simulink model "Project"  (R2019a)
settings: Solver=VariableStepAuto  StartTime=0.0  StopTime=9  RelTol=1e-3
model workspace (MAT data in the model file):
  tc = 0.05
libraries: Solver_SF x2, simulink x2
settings Model: Creator=admin  LastModifiedBy=Chuan
settings DataIOCC: ReturnWorkspaceOutputs=off

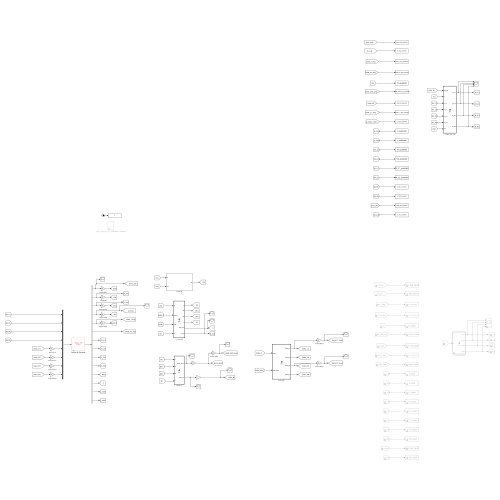
[thumbnail: Simulink's stored preview of the top-level diagram]
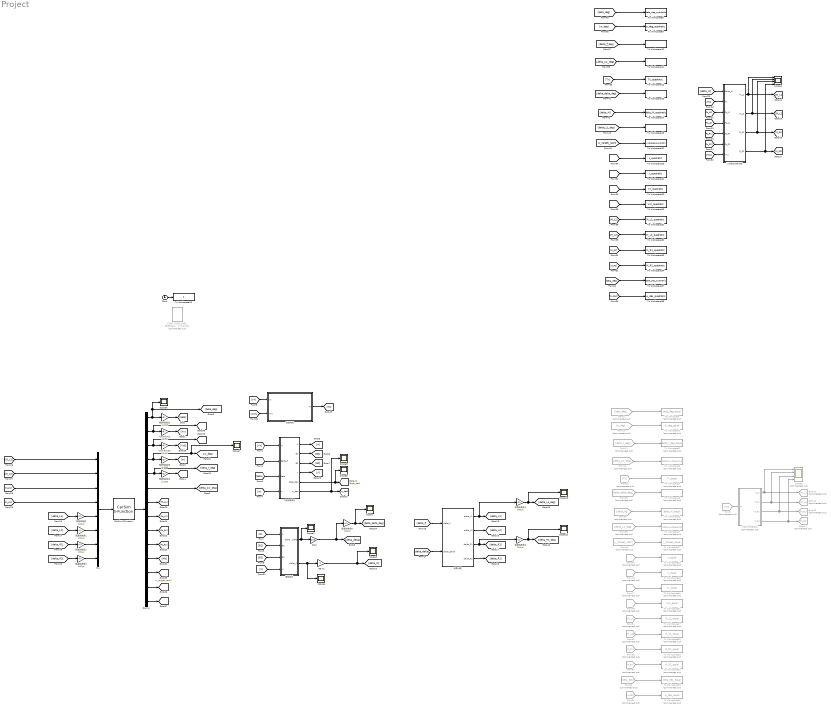
== system Project ==
  CarSim S-Function : Solver_SF/CarSim S-Function  Priority=1  SIMFILE=simfile.sim
  Clock : Clock
  Demux : Demux  Outputs=14
  From10 : From  Commented=on  GotoTag=w_deg
  From11 : From  Commented=on  GotoTag=delta_f_deg
  From12 : From  Commented=on  GotoTag=delta_sw_deg
  From15 : From  Commented=on  GotoTag=Tx
  From2 : From  Commented=on  GotoTag=beta_deg
  From33 : From  Commented=on  GotoTag=delta_delta_deg
  From34 : From  Commented=on  GotoTag=delta_M
  From35 : From  Commented=on  GotoTag=delta_L1_deg
  From44 : From  Commented=on  GotoTag=y_target_nash
  From45 : From  Commented=on  GotoTag=x_nash
  From46 : From  Commented=on  GotoTag=y_nash
  From47 : From  Commented=on  GotoTag=Vx_km
  From48 : From  Commented=on  GotoTag=Vxt_km
  From54 : From  Commented=on  GotoTag=M_L1
  From55 : From  Commented=on  GotoTag=M_L2
  From56 : From  Commented=on  GotoTag=M_R1
  From57 : From  Commented=on  GotoTag=M_R2
  From62 : From  Commented=on  GotoTag=beta_des
  From63 : From  Commented=on  GotoTag=w_des
  From9 : From  Commented=on  GotoTag=Tx
  Gain : Gain  Gain=1/10
  Gain1 : Gain
  Goto11 : Goto  Commented=on  GotoTag=M_L1
  Goto12 : Goto  Commented=on  GotoTag=M_L2
  Goto13 : Goto  Commented=on  GotoTag=M_R1
  Goto14 : Goto  Commented=on  GotoTag=M_R2
  Mux : Mux  Inputs=8
  Scope{,2..4,6..11} (10 alike) : Scope
  Scope1 : Scope  NumInputPorts=4
  Scope5 : Scope  Commented=on  NumInputPorts=4
  To Workspace : ToWorkspace  Commented=on  VariableName=beta_deg_equal  SampleTime=-1
  To Workspace1 : ToWorkspace  Commented=on  VariableName=w_deg_equal  SampleTime=-1
  To Workspace10 : ToWorkspace  VariableName=delta_f_deg_quadratic  SampleTime=-1
  To Workspace11 : ToWorkspace  VariableName=delta_sw_deg_quadratic  SampleTime=-1
  To Workspace12 : ToWorkspace  VariableName=Tx_quadratic  SampleTime=-1
  To Workspace13 : ToWorkspace  VariableName=delta_delta_deg_quadratic  SampleTime=-1
  To Workspace14 : ToWorkspace  VariableName=delta_M_quadratic  SampleTime=-1
  To Workspace15 : ToWorkspace  VariableName=delta_L1_deg_quadratic  SampleTime=-1
  To Workspace16 : ToWorkspace  VariableName=t  SampleTime=-1
  To Workspace17 : ToWorkspace  Commented=on  VariableName=y_target_equal  SampleTime=-1
  To Workspace18 : ToWorkspace  Commented=on  VariableName=x_equal  SampleTime=-1
  To Workspace19 : ToWorkspace  Commented=on  VariableName=y_equal  SampleTime=-1
  To Workspace2 : ToWorkspace  Commented=on  VariableName=delta_f_deg_equal  SampleTime=-1
  To Workspace20 : ToWorkspace  Commented=on  VariableName=Vx_equal  SampleTime=-1
  To Workspace21 : ToWorkspace  Commented=on  VariableName=Vxt_equal  SampleTime=-1
  To Workspace22 : ToWorkspace  VariableName=y_target_quadratic  SampleTime=-1
  To Workspace23 : ToWorkspace  VariableName=x_quadratic  SampleTime=-1
  To Workspace24 : ToWorkspace  VariableName=y_quadratic  SampleTime=-1
  To Workspace25 : ToWorkspace  VariableName=Vx_quadratic  SampleTime=-1
  To Workspace26 : ToWorkspace  VariableName=Vxt_quadratic  SampleTime=-1
  To Workspace27 : ToWorkspace  Commented=on  VariableName=M_L1_equal  SampleTime=-1
  To Workspace28 : ToWorkspace  Commented=on  VariableName=M_L2_equal  SampleTime=-1
  To Workspace29 : ToWorkspace  Commented=on  VariableName=M_R1_equal  SampleTime=-1
  To Workspace3 : ToWorkspace  Commented=on  VariableName=delta_sw_deg_equal  SampleTime=-1
  To Workspace30 : ToWorkspace  Commented=on  VariableName=M_R2_equal  SampleTime=-1
  To Workspace31 : ToWorkspace  VariableName=M_L1_quadratic  SampleTime=-1
  To Workspace32 : ToWorkspace  VariableName=M_L2_quadratic  SampleTime=-1
  To Workspace33 : ToWorkspace  VariableName=M_R1_quadratic  SampleTime=-1
  To Workspace34 : ToWorkspace  VariableName=M_R2_quadratic  SampleTime=-1
  To Workspace35 : ToWorkspace  Commented=on  VariableName=beta_des_equal  SampleTime=-1
  To Workspace36 : ToWorkspace  Commented=on  VariableName=w_des_equal  SampleTime=-1
  To Workspace37 : ToWorkspace  VariableName=beta_des_quadratic  SampleTime=-1
  To Workspace38 : ToWorkspace  VariableName=w_des_quadratic  SampleTime=-1
  To Workspace4 : ToWorkspace  Commented=on  VariableName=Tx_equal  SampleTime=-1
  To Workspace5 : ToWorkspace  Commented=on  VariableName=delta_delta_deg_equal  SampleTime=-1
  To Workspace6 : ToWorkspace  Commented=on  VariableName=delta_M_equal  SampleTime=-1
  To Workspace7 : ToWorkspace  Commented=on  VariableName=delta_L1_deg_equal  SampleTime=-1
  To Workspace8 : ToWorkspace  VariableName=beta_deg_quadratic  SampleTime=-1
  To Workspace9 : ToWorkspace  VariableName=w_deg_quadratic  SampleTime=-1
  km/h转m/s : Gain  Gain=10/36
  km/h转m/s1 : Gain  Gain=10/36
  二次规划力矩分配 : MATLAB Function  TreatAsAtomicUnit=on
  二自由度部分 : MATLAB Function  TreatAsAtomicUnit=on
  力矩平均分配测试 : MATLAB Function  Commented=on  TreatAsAtomicUnit=on
  博弈部分 : MATLAB Function  TreatAsAtomicUnit=on
  弧度转角度{,1..6} (7 alike) : Gain  Gain=180/pi
  无控制_无博弈及分配_需调整carsim为nocontrol : Subsystem  Commented=on
  角度转弧度1 : Gain  Gain=pi/180
  角度转弧度2 : Gain  Gain=pi/180
  角度转弧度3 : Gain  Gain=pi/180
  转角分配 : MATLAB Function  TreatAsAtomicUnit=on
  轮毂电机 : Subsystem
  wires:
  [B1] -> 博弈部分/2(B1)
  转角分配/4(delta_R2) -> [delta_R2]
  [delta_delta] -> 转角分配/2(delta_delta)
  博弈部分/1(delta_delta) -> Gain/1, Scope2/1
  [delta_R1] -> 弧度转角度2/1
  二自由度部分/1(A) -> [A]
  [A] -> 博弈部分/1(A)
  [w] -> 二自由度部分/4(w)
  [delta_f] -> 二自由度部分/2(delta_f)
  Demux/4 -> Scope7/1, [w_deg], 角度转弧度3/1
  [delta_R2] -> 弧度转角度3/1
  Demux/3 -> [Vxt_km], km/h转m/s1/1
  [B2] -> 博弈部分/3(B2)
  Demux/7 -> [Fz_L1]
  弧度转角度/1 -> Mux/5
  [Vx] -> 二自由度部分/1(Vx)
  [delta_f] -> 转角分配/1(delta_f)
  二自由度部分/2(B1) -> [B1]
  二自由度部分/4(X) -> [X]
  角度转弧度1/1 -> [beta]
  Demux/2 -> [Vx_km], km/h转m/s/1
  [X] -> 博弈部分/4(X)
  [Vxt] -> 轮毂电机/2(Vxt)
  [Vx] -> 轮毂电机/1(Vx)
  [delta_L1] -> 弧度转角度/1
  弧度转角度2/1 -> Mux/7
  [M_L1] -> Mux/1
  [M_R1] -> Mux/3
  轮毂电机/1(Tx) -> [Tx]
  Demux/10 -> [Fz_R2]
  [delta_L2] -> 弧度转角度1/1
  角度转弧度2/1 -> [delta_f]
  博弈部分/2(delta_M) -> Gain1/1, Scope4/1
  角度转弧度3/1 -> [w]
  转角分配/3(delta_R1) -> 弧度转角度6/1, [delta_R1]
  Demux/1 -> Scope6/1, [beta_deg], 角度转弧度1/1
  弧度转角度3/1 -> Mux/8
  弧度转角度1/1 -> Mux/6
  Demux/8 -> [Fz_L2]
  Demux/5 -> [delta_f_deg], 角度转弧度2/1
  Mux/1 -> CarSim S-Function/1
  [beta] -> 二自由度部分/3(beta)
  Demux/9 -> [Fz_R1]
  CarSim S-Function/1 -> Demux/1
  二自由度部分/3(B2) -> [B2]
  [M_L2] -> Mux/2
  [M_R2] -> Mux/4
  Demux/11 -> [Mu]
  km/h转m/s1/1 -> [Vxt]
  转角分配/1(delta_L1) -> 弧度转角度4/1, [delta_L1]
  km/h转m/s/1 -> [Vx]
  [Fz_L2] -> 二次规划力矩分配/4(Fz_L2)
  [Tx] -> 二次规划力矩分配/2(Tx)
  二次规划力矩分配/4(M_R2) -> Scope1/4, [M_R2]
  二次规划力矩分配/1(M_L1) -> Scope1/1, [M_L1]
  [Fz_L1] -> 二次规划力矩分配/3(Fz_L1)
  [Fz_R1] -> 二次规划力矩分配/5(Fz_R1)
  [Mu] -> 二次规划力矩分配/7(miu)
  二次规划力矩分配/3(M_R1) -> Scope1/3, [M_R1]
  二次规划力矩分配/2(M_L2) -> Scope1/2, [M_L2]
  [Fz_R2] -> 二次规划力矩分配/6(Fz_R2)
  [delta_M] -> 二次规划力矩分配/1(delta_M)
  力矩平均分配测试/1(M_L1) -> Scope5/1, Goto11/1
  From9/1 -> 力矩平均分配测试/1(Tx)
  力矩平均分配测试/3(M_R1) -> Scope5/3, Goto13/1
  力矩平均分配测试/2(M_L2) -> Scope5/2, Goto12/1
  力矩平均分配测试/4(M_R2) -> Scope5/4, Goto14/1
  Demux/6 -> [delta_sw_deg]
  弧度转角度4/1 -> Scope10/1, [delta_L1_deg]
  弧度转角度5/1 -> Scope/1, [delta_delta_deg]
  Gain/1 -> 弧度转角度5/1, [delta_delta]
  From2/1 -> To Workspace/1
  From10/1 -> To Workspace1/1
  From11/1 -> To Workspace2/1
  From12/1 -> To Workspace3/1
  From15/1 -> To Workspace4/1
  From33/1 -> To Workspace5/1
  From34/1 -> To Workspace6/1
  From35/1 -> To Workspace7/1
  [delta_L1_deg] -> To Workspace15/1
  [delta_M] -> To Workspace14/1
  [delta_delta_deg] -> To Workspace13/1
  [Tx] -> To Workspace12/1
  [delta_sw_deg] -> To Workspace11/1
  [delta_f_deg] -> To Workspace10/1
  [w_deg] -> To Workspace9/1
  [beta_deg] -> To Workspace8/1
  Clock/1 -> To Workspace16/1
  Demux/12 -> [y_target_nash]
  Demux/14 -> [y_nash]
  Demux/13 -> [x_nash]
  From44/1 -> To Workspace17/1
  From45/1 -> To Workspace18/1
  From46/1 -> To Workspace19/1
  From47/1 -> To Workspace20/1
  From48/1 -> To Workspace21/1
  [Vx_km] -> To Workspace25/1
  [Vxt_km] -> To Workspace26/1
  [y_target_nash] -> To Workspace22/1
  [x_nash] -> To Workspace23/1
  [y_nash] -> To Workspace24/1
  From57/1 -> To Workspace30/1
  From56/1 -> To Workspace29/1
  From55/1 -> To Workspace28/1
  From54/1 -> To Workspace27/1
  [M_R1] -> To Workspace33/1
  [M_L2] -> To Workspace32/1
  [M_L1] -> To Workspace31/1
  [M_R2] -> To Workspace34/1
  Gain1/1 -> Scope3/1, [delta_M]
  二自由度部分/6(w_des) -> Scope9/1, [w_des]
  弧度转角度6/1 -> [delta_R1_deg], Scope11/1
  转角分配/2(delta_L2) -> [delta_L2]
  From62/1 -> To Workspace35/1
  From63/1 -> To Workspace36/1
  [w_des] -> To Workspace38/1
  [beta_des] -> To Workspace37/1
  二自由度部分/5(beta_des) -> Scope8/1, [beta_des]

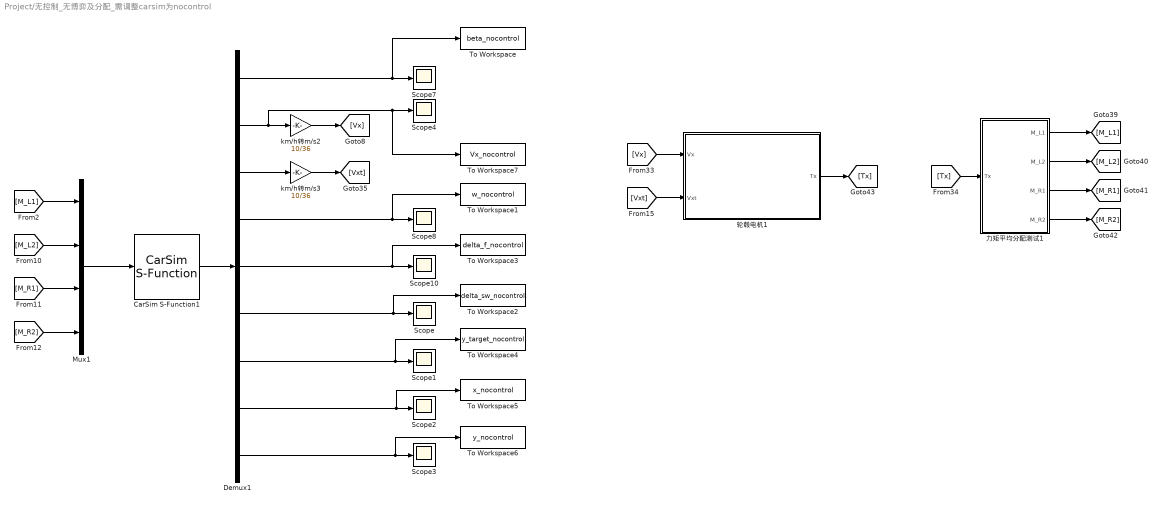
== system Project/无控制_无博弈及分配_需调整carsim为nocontrol ==
  CarSim S-Function1 : Solver_SF/CarSim S-Function  Priority=1  SIMFILE=simfile.sim
  Demux1 : Demux  Outputs=9
  Mux1 : Mux
  Scope{,1..4,7..8,10} (8 alike) : Scope
  To Workspace : ToWorkspace  VariableName=beta_nocontrol  SampleTime=-1
  To Workspace1 : ToWorkspace  VariableName=w_nocontrol  SampleTime=-1
  To Workspace2 : ToWorkspace  VariableName=delta_sw_nocontrol  SampleTime=-1
  To Workspace3 : ToWorkspace  VariableName=delta_f_nocontrol  SampleTime=-1
  To Workspace4 : ToWorkspace  VariableName=y_target_nocontrol  SampleTime=-1
  To Workspace5 : ToWorkspace  VariableName=x_nocontrol  SampleTime=-1
  To Workspace6 : ToWorkspace  VariableName=y_nocontrol  SampleTime=-1
  To Workspace7 : ToWorkspace  VariableName=Vx_nocontrol  SampleTime=-1
  km/h转m/s2 : Gain  Gain=10/36
  km/h转m/s3 : Gain  Gain=10/36
  力矩平均分配测试1 : MATLAB Function  TreatAsAtomicUnit=on
  轮毂电机1 : Subsystem
  wires:
  Mux1/1 -> CarSim S-Function1/1
  [Vxt] -> 轮毂电机1/2(Vxt)
  Demux1/3 -> km/h转m/s3/1
  CarSim S-Function1/1 -> Demux1/1
  [M_R2] -> Mux1/4
  km/h转m/s2/1 -> [Vx]
  [M_L2] -> Mux1/2
  Demux1/5 -> To Workspace3/1, Scope10/1
  [Tx] -> 力矩平均分配测试1/1(Tx)
  [M_R1] -> Mux1/3
  Demux1/4 -> To Workspace1/1, Scope8/1
  力矩平均分配测试1/2(M_L2) -> [M_L2]
  力矩平均分配测试1/1(M_L1) -> [M_L1]
  轮毂电机1/1(Tx) -> [Tx]
  km/h转m/s3/1 -> [Vxt]
  [M_L1] -> Mux1/1
  力矩平均分配测试1/4(M_R2) -> [M_R2]
  [Vx] -> 轮毂电机1/1(Vx)
  力矩平均分配测试1/3(M_R1) -> [M_R1]
  Demux1/1 -> To Workspace/1, Scope7/1
  Demux1/6 -> To Workspace2/1, Scope/1
  Demux1/7 -> To Workspace4/1, Scope1/1
  Demux1/8 -> To Workspace5/1, Scope2/1
  Demux1/9 -> To Workspace6/1, Scope3/1
  Demux1/2 -> To Workspace7/1, Scope4/1, km/h转m/s2/1

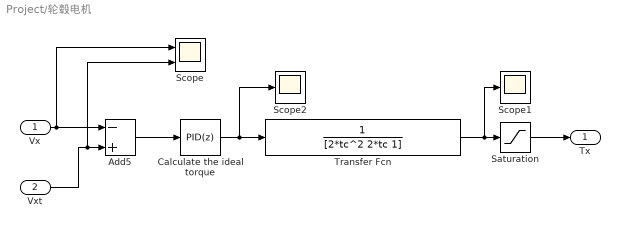
== system Project/轮毂电机 ==
  Vx : Inport
  Vxt : Inport  Port=2
  Add5 : Sum  Inputs=-+
  Calculate the ideal torque : simulink/Continuous/PID Controller  Controller=PID  Form=Parallel  TimeDomain=Discrete-time  SampleTime=-1  IntegratorMethod=Forward Euler  FilterMethod=Forward Euler  ControllerParametersSource=internal  P=500  I=500  D=10  UseFilter=on  N=100  TunerSelectOption=Transfer Function Based (PID Tuner App)  InitialConditionSource=internal  InitialConditionForIntegrator=0  InitialConditionForFilter=0  DifferentiatorICPrevScaledInput=0  ExternalReset=none  TrackingMode=off  Kt=1  LimitOutput=off  UpperSaturationLimit=inf  LowerSaturationLimit=-inf  LinearizeAsGain=off  AntiWindupMode=none  Kb=1  POutMin=[]  POutMax=[]  IOutMin=[]  IOutMax=[]  DOutMin=[]  DOutMax=[]  NOutMin=[]  NOutMax=[]  SumOutMin=[]  SumOutMax=[]  SaturationOutMin=[]  SaturationOutMax=[]  PParamMin=[]  PParamMax=[]  IParamMin=[]  IParamMax=[]  DParamMin=[]  DParamMax=[]  NParamMin=[]  NParamMax=[]  KbParamMin=[]  KbParamMax=[]  KtParamMin=[]  KtParamMax=[]  KbOutMin=[]  KbOutMax=[]  KtOutMin=[]  KtOutMax=[]  IntegratorOutMin=[]  IntegratorOutMax=[]  FilterOutMin=[]  FilterOutMax=[]  SumI1OutMin=[]  SumI1OutMax=[]  SumI2OutMin=[]  SumI2OutMax=[]  SumI3OutMin=[]  SumI3OutMax=[]  SumI4OutMin=[]  SumI4OutMax=[]  SumDOutMin=[]  SumDOutMax=[]  DifferentiatorOutMin=[]  DifferentiatorOutMax=[]  FilterDiffOutCoefMin=[]  FilterDiffOutCoefMax=[]  ReciprocalOutMin=[]  ReciprocalOutMax=[]  SumDenOutMin=[]  SumDenOutMax=[]  SumNumOutMin=[]  SumNumOutMax=[]  DivideOutMin=[]  DivideOutMax=[]  IntegratorContinuousStateAttributes=''  IntegratorStateMustResolveToSignalObject=off  IntegratorRTWStateStorageClass=Auto  FilterContinuousStateAttributes=''  FilterStateMustResolveToSignalObject=off  FilterRTWStateStorageClass=Auto  ParallelPVariant=InternalParameters  IdealPVariant=Disabled  IVariant=InternalParameters  DVariant=InternalParameters  IntegratorVariant=Discrete  SatVariant=Disabled  AWVariant=Passthrough  PCopyVariant=Disabled  TRVariant=Disabled  FdbkBlocksVariant=Forward  IdealPFdbkVariant=Disabled  SatFdbkVariant=Disabled  DerivativeFilterVariant=ForwardEulerFilter  NVariant=InternalParameters  NCopyVariant=Disabled  FilterICVariant=InternalICsFilter  IntegratorICVariant=InternalICs  ExternalResetVariant=Disabled  TRSumVariant=Passthrough  SumFdbkVariant=Disabled  SumVariant=Sum_PID
  Saturation : Saturate  UpperLimit=319  LowerLimit=-319
  Scope : Scope  NumInputPorts=2
  Scope1 : Scope
  Scope2 : Scope
  Transfer Fcn : TransferFcn  Denominator=[2*tc^2 2*tc 1]
  Tx : Outport
  wires:
  Vxt/1 -> Scope/2, Add5/2
  Vx/1 -> Scope/1, Add5/1
  Add5/1 -> Calculate the ideal torque/1
  Calculate the ideal torque/1 -> Scope2/1, Transfer Fcn/1
  Transfer Fcn/1 -> Scope1/1, Saturation/1
  Saturation/1 -> Tx/1

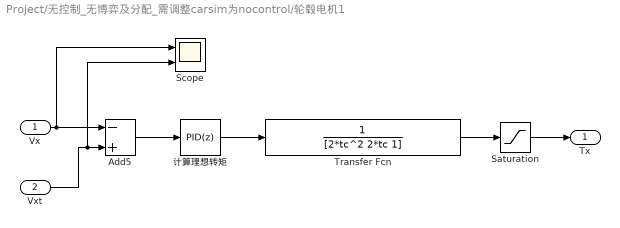
== system Project/无控制_无博弈及分配_需调整carsim为nocontrol/轮毂电机1 ==
  Vx : Inport
  Vxt : Inport  Port=2
  Add5 : Sum  Inputs=-+
  Saturation : Saturate  UpperLimit=319  LowerLimit=-319
  Scope : Scope  NumInputPorts=2
  Transfer Fcn : TransferFcn  Denominator=[2*tc^2 2*tc 1]
  计算理想转矩 : simulink/Continuous/PID Controller  Controller=PID  Form=Parallel  TimeDomain=Discrete-time  SampleTime=-1  IntegratorMethod=Forward Euler  ControllerParametersSource=internal  P=500  I=500  D=10  N=100  UseFilter=on  TunerSelectOption=Transfer Function Based (PID Tuner App)  InitialConditionSource=internal  InitialConditionForIntegrator=0  InitialConditionForFilter=0  DifferentiatorICPrevScaledInput=0  ExternalReset=none  TrackingMode=off  Kt=1  LimitOutput=off  UpperSaturationLimit=inf  LowerSaturationLimit=-inf  LinearizeAsGain=off  AntiWindupMode=none  Kb=1  POutMin=[]  POutMax=[]  IOutMin=[]  IOutMax=[]  DOutMin=[]  DOutMax=[]  NOutMin=[]  NOutMax=[]  SumOutMin=[]  SumOutMax=[]  SaturationOutMin=[]  SaturationOutMax=[]  PParamMin=[]  PParamMax=[]  IParamMin=[]  IParamMax=[]  DParamMin=[]  DParamMax=[]  NParamMin=[]  NParamMax=[]  KbParamMin=[]  KbParamMax=[]  KtParamMin=[]  KtParamMax=[]  KbOutMin=[]  KbOutMax=[]  KtOutMin=[]  KtOutMax=[]  IntegratorOutMin=[]  IntegratorOutMax=[]  FilterOutMin=[]  FilterOutMax=[]  SumI1OutMin=[]  SumI1OutMax=[]  SumI2OutMin=[]  SumI2OutMax=[]  SumI3OutMin=[]  SumI3OutMax=[]  SumI4OutMin=[]  SumI4OutMax=[]  SumDOutMin=[]  SumDOutMax=[]  DifferentiatorOutMin=[]  DifferentiatorOutMax=[]  FilterDiffOutCoefMin=[]  FilterDiffOutCoefMax=[]  ReciprocalOutMin=[]  ReciprocalOutMax=[]  SumDenOutMin=[]  SumDenOutMax=[]  SumNumOutMin=[]  SumNumOutMax=[]  DivideOutMin=[]  DivideOutMax=[]  IntegratorContinuousStateAttributes=''  IntegratorStateMustResolveToSignalObject=off  IntegratorRTWStateStorageClass=Auto  FilterContinuousStateAttributes=''  FilterStateMustResolveToSignalObject=off  FilterRTWStateStorageClass=Auto  ParallelPVariant=InternalParameters  IdealPVariant=Disabled  IVariant=InternalParameters  DVariant=InternalParameters  IntegratorVariant=Discrete  SatVariant=Disabled  AWVariant=Passthrough  PCopyVariant=Disabled  TRVariant=Disabled  FdbkBlocksVariant=Forward  IdealPFdbkVariant=Disabled  SatFdbkVariant=Disabled  DerivativeFilterVariant=ForwardEulerFilter  NVariant=InternalParameters  NCopyVariant=Disabled  FilterICVariant=InternalICsFilter  IntegratorICVariant=InternalICs  ExternalResetVariant=Disabled  TRSumVariant=Passthrough  SumFdbkVariant=Disabled  SumVariant=Sum_PID
  Tx : Outport
  wires:
  Saturation/1 -> Tx/1
  Transfer Fcn/1 -> Saturation/1
  计算理想转矩/1 -> Transfer Fcn/1
  Add5/1 -> 计算理想转矩/1
  Vx/1 -> Add5/1, Scope/1
  Vxt/1 -> Add5/2, Scope/2

== matlab function Project/二次规划力矩分配 ==
  data: delta_M input; Tx input; Fz_L1 input; Fz_L2 input; Fz_R1 input; Fz_R2 input; M_L1 output; M_L2 output; M_R1 output; M_R2 output; miu input
function [M_L1, M_L2, M_R1, M_R2] = fcn(delta_M, Tx, Fz_L1, Fz_L2, Fz_R1, Fz_R2, miu)
%调用外部函数
coder.extrinsic('quadprog');
%%
%基本参数
R = 0.5752;%单位：米
t = 1.695;%轮距
Tmmax = 319;%峰值转矩
%%
if(delta_M == 0)
    M_L1 = Tx;M_L2 = Tx;M_R1 = Tx;M_R2 = Tx;
else
    %%
    % QP矩阵参数
    % 目标方程参数
        H11 = 2/((delta_M*Fz_L1)^2*R^2);
        H22 = 2/((delta_M*Fz_L2)^2*R^2);
        H33 = 2/((delta_M*Fz_R1)^2*R^2);
        H44 = 2/((delta_M*Fz_R2)^2*R^2);
        
        H = diag([H11 H22 H33 H44]);
    %不等式约束
        A = [];
        b = [];
    %等式约束
        Aeq = [1 1 1 1 ; -1 1 1 -1];
        Beq = [Tx*4 ; 2*R*delta_M/t];
    %上下限约束
        LB = [0;0;0;0];
        UB = [min(Tmmax,(miu*Fz_L1*R)) ; min(Tmmax,(miu*Fz_L2*R)) ; min(Tmmax,(miu*Fz_R1*R)) ; min(Tmmax,(miu*Fz_R2*R)) ];
    % 求解二次规划
        X = quadprog(H,[],A,b,Aeq,Beq,LB,UB);
    %分配
        M_L1 = X(1,1);
        M_L2 = X(2,1);
        M_R1 = X(3,1);
        M_R2 = X(4,1);
end

== matlab function Project/力矩平均分配测试 ==
  data: Tx input; M_L1 output; M_L2 output; M_R1 output; M_R2 output
function [M_L1,M_L2, M_R1, M_R2] = fcn(Tx)

M_L1 = Tx/4;
M_L2 = Tx/4;
M_R1 = Tx/4;
M_R2 = Tx/4;

== matlab function Project/无控制_无博弈及分配_需调整carsim为nocontrol/力矩平均分配测试1 ==
  data: Tx input; M_L1 output; M_L2 output; M_R1 output; M_R2 output
function [M_L1,M_L2, M_R1, M_R2] = fcn(Tx)

M_L1 = Tx/4;
M_L2 = Tx/4;
M_R1 = Tx/4;
M_R2 = Tx/4;

== matlab function Project/二自由度部分 ==
  data: Vx input; delta_f input; A output; B1 output; B2 output; beta input; w input; X output; beta_des output; w_des output
function [A,B1,B2,X,beta_des,w_des] = fcn( Vx ,  delta_f, beta, w)

    %%
    % 基本参数
    kf = 82000;%前轴轮胎侧偏刚度
    kr = 130000;%后轴轮胎侧偏刚度
    m = 1020;%整车质量
    a = 1.165;%前轴距(m)
    b = 2.33-1.165;%后轴距(m)
    L = 2.33;
    Iz = 1020;%整车横摆转动惯量
    
    %%
    % 状态方程参数计算
    a11 = -(kf+kr)/(m*Vx);
    a12 = (-a*kf+b*kr)/(m*Vx^2)-1;
    a21 = (-a*kf+b*kr)/Iz;
    a22 = (-kf*a^2-kr*b^2)/(Iz*Vx);
    A = [a11 a12 ; a21 a22];%状态方程中的A
    
    b_1_11 = kf/(m*Vx);
    b_1_21 = a*kf/Iz;
    B1 = [b_1_11;b_1_21];%状态方程中的B1
    
    b_2_11 = 0;
    b_2_21 = 1/Iz;
    B2 = [b_2_11;b_2_21];%状态方程中的B2
    %%
    %理想参数
    Kus = m*(a/kr-b/kf)/(L^2*a*b);
    w_des = Vx*delta_f  /  (L*(1+Kus*Vx^2));
    beta_des = (b-a*m*Vx^2/(kr*L))*delta_f  /  (L*(1+Kus*Vx^2));
    %%
    delta_beta = beta - beta_des;
    delta_w = w - w_des;
    X = [delta_beta ; delta_w];

== matlab function Project/博弈部分 ==
  data: A input; delta_delta output; B1 input; B2 input; delta_M output; X input
function [delta_delta,delta_M] = fcn(A, B1, B2, X)
%调用外部函数
coder.extrinsic('are');
    delta_delta = 0;
    delta_M = 0;

    %%
    %权重系数
    v1 = [1000000 1000];
    Q1 = diag(v1);%AFS 系统的权重矩阵
    v2 = [1000000 1000];
    Q2 = diag(v2);%DYC 系统的权重矩阵
    R11 = 50000;%AFS前轮转向权重矩阵
    R22 = 0.001;%DYC横摆力矩权重矩阵
    R12 = 0.000001;% ΔM 对AFS 的影响权重矩阵
    R21 = 0.000001;% Δδ 对 DYC 的影响权重矩阵
    %方程所需参数
    S11 = B1*(R11^(-1))*R11*(R11^(-1))*B1';
    S12 = B2*(R22^(-1))*R12*(R22^(-1))*B2';
    S21 = B1*(R11^(-1))*R21*(R11^(-1))*B1';
    S22 = B2*(R22^(-1))*R22*(R22^(-1))*B2';
    %%
    %初始值计算
    K1_0 = [1 1 ; 1 1];K2_0 = [1 1 ; 1 1];%定义变量格式，防止报错
    K1_0 = are(A,S11,Q1);
    K2_0 = are(A,S22,Q2);
    %%
    %博弈迭代过程
    
    epslion = exp(-5);
    K1_1 = [1 1 ; 1 1];K2_1 = [1 1 ; 1 1];%定义变量格式，防止报错
    
    while(1)
        %1号方程求解
        A_1 = A-S22*K2_0;
        Q1_1 = Q1+K2_0*S12*K2_0;
        K1_1 = are(A_1,S11,Q1_1);
        %2号方程求解
        A_2 = A-S11*K1_0;
        Q2_1 = Q2+K1_0*S21*K1_0;
        K2_1 = are(A_2,S22,Q2_1);
        %循环条件
        if (norm(K1_1-K1_0) < epslion  && norm(K2_1-K2_0) < epslion)
            break;
        else
            K1_0 = K1_1;
            K2_0 = K2_1;
        end
        %%
        %求解输出数据
        delta_delta = -(R11)^(-1)*B1'*K1_1*X;
        delta_M = -(R22)^(-1)*B2'*K2_1*X;
    end

== matlab function Project/转角分配 ==
  data: delta_f input; delta_L1 output; delta_delta input; delta_L2 output; delta_R1 output; delta_R2 output
function [delta_L1,delta_L2, delta_R1, delta_R2] = fcn(delta_f, delta_delta)
%%
%后轮基本参数
% delta_r = k*delta_f;
%前轮
% if (delta_delta>1*pi/180 || delta_delta<-1*pi/180)
%     delta_L1 = delta_f + 5*pi/180; %弧度制分配
%     delta_R1 = delta_L1;%为了方便控制，假设同轴左右轮转角大小相等
% else
    delta_L1 = delta_f + delta_delta; %弧度制分配
    delta_R1 = delta_L1;%为了方便控制，假设同轴左右轮转角大小相等

%%
%后轮
%delta_delta_r = k*delta_delta;%后轮转角变化值
%delta_L2 = delta_r + delta_delta_r ;%弧度制分配
%delta_R2 = delta_L2 ;%为了方便控制，假设同轴左右轮转角大小相等

delta_R2 = 0;
delta_L2 = 0;
